simulink model "Gorev3"  (R2019a)
settings: Solver=ode45  StartTime=0.0  StopTime=10.0  RelTol=1e-5
libraries: simulink x1
settings Model: Creator=handeyildirim  LastModifiedBy=handeyildirim

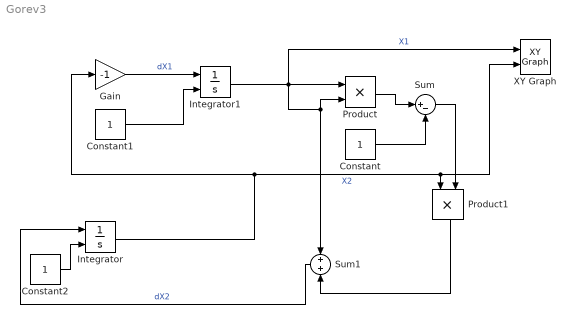
== system Gorev3 ==
  Constant : Constant
  Constant1 : Constant
  Constant2 : Constant
  Gain : Gain  Gain=-1
  Integrator : Integrator  InitialConditionSource=external
  Integrator1 : Integrator  InitialConditionSource=external
  Product : Product
  Product1 : Product
  Sum : Sum  Inputs=|+-
  Sum1 : Sum
  XY Graph : simulink/Sinks/XY Graph  xmin=-0.6  xmax=1.1  ymin=-0.4  ymax=1.2  st=0.2
  wires:
  Integrator1/1 -> XY Graph/1, Sum1/1, Product/2, Product/1  "X1"
  Sum1/1 -> Integrator/1  "dX2"
  Integrator/1 -> Gain/1, XY Graph/2, Product1/1  "X2"
  Gain/1 -> Integrator1/1  "dX1"
  Constant/1 -> Sum/2
  Product/1 -> Sum/1
  Sum/1 -> Product1/2
  Product1/1 -> Sum1/2
  Constant1/1 -> Integrator1/2
  Constant2/1 -> Integrator/2
